simulink library "mbed_targets_stm_nucleo_f303k8"  (R2015a)
settings: Solver=ode45  StartTime=0.0  StopTime=10.0  RelTol=1e-3
libraries: mbed_lib x5
settings Model: CovSFcnEnable=off  Creator=oh  LastModifiedBy=oh
settings DebuggingCC: SolverPrmCheckMsg=warning

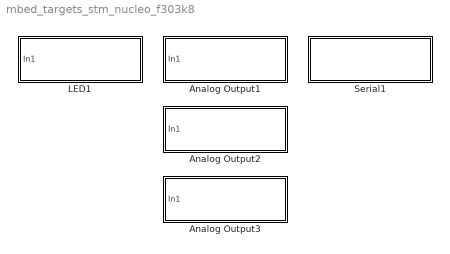
== system mbed_targets_stm_nucleo_f303k8 ==
  Analog Output1 : Subsystem  mask{Parameter1=0}
      mask Display:
      | offset=0.7;
      | plot([0+offset:0.025:0.25+offset],0.3*sin(2*pi*[0:0.1:1])+0.5)
      | port_label('input',1,['DAC1_1 (PA_4)']);
  Analog Output2 : Subsystem  mask{Parameter1=0}
      mask Display:
      | offset=0.7;
      | plot([0+offset:0.025:0.25+offset],0.3*sin(2*pi*[0:0.1:1])+0.5)
      | port_label('input',1,['DAC1_2 (PA_5)']);
  Analog Output3 : Subsystem  mask{Parameter1=0}
      mask Display:
      | offset=0.7;
      | plot([0+offset:0.025:0.25+offset],0.3*sin(2*pi*[0:0.1:1])+0.5)
      | port_label('input',1,['DAC2_1 (PA_6)']);
  LED1 : Subsystem  mask{Parameter1=0}
      mask Display:
      | plot([0.5 0.65 0.65 0.85 0.85 1],[0.3 0.3 0.7 0.7 0.3 0.3])
      | port_label('input',1,['LED1']);
  Serial1 : Subsystem  mask(mbed Serial Configuration){Parameter1=0, BaudRate=9600}
      mask prompts: BaudRate "Baud Rate:"
      mask help:
      | This blocks sets up the serial connection over ST-Link on the NUCLEO_F303 mbed board. You must have one of these blocks in any model that ues the Serial Write or Serial Read blocks.
      |
      | Set the baud rate to match the device that you are communicating with. Standard rates include:300, 1200, 2400, 4800, 9600, 14400, 19200, 28800, 38400, 57600, or 115200.
      mask TypeOptions BaudRate: Serial Configuration/BaudRate
      mask Display: disp(['Serial1(USB)\nTX:PA_2, RX:PA_15'])

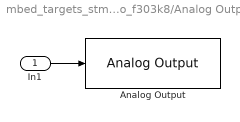
== system mbed_targets_stm_nucleo_f303k8/Analog Output1 ==
  In1 : Inport
  Analog Output : mbed_lib/GPIO/Analog Output  SParameter2=A  SParameter1=4  inputVariant=Double: 0 - 1.0f  SampleTime=-1
  wires:
  In1/1 -> Analog Output/1

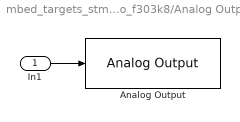
== system mbed_targets_stm_nucleo_f303k8/Analog Output2 ==
  In1 : Inport
  Analog Output : mbed_lib/GPIO/Analog Output  SParameter2=A  SParameter1=5  inputVariant=Double: 0 - 1.0f  SampleTime=-1
  wires:
  In1/1 -> Analog Output/1

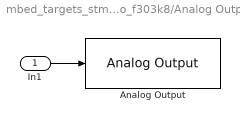
== system mbed_targets_stm_nucleo_f303k8/Analog Output3 ==
  In1 : Inport
  Analog Output : mbed_lib/GPIO/Analog Output  SParameter2=A  SParameter1=6  inputVariant=Double: 0 - 1.0f  SampleTime=-1
  wires:
  In1/1 -> Analog Output/1

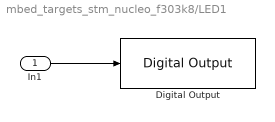
== system mbed_targets_stm_nucleo_f303k8/LED1 ==
  In1 : Inport
  Digital Output : mbed_lib/GPIO/Digital Output  SParameter2=B  SParameter1=3  SParameter3=PullDefault  SampleTime=-1
  wires:
  In1/1 -> Digital Output/1

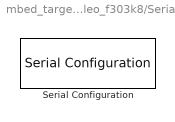
== system mbed_targets_stm_nucleo_f303k8/Serial1 ==
  Serial Configuration : mbed_lib/Serial/Serial Configuration  SerialPort=1  TXPort=A  TXPin=2  RXPort=A  RXPin=15  BaudRate=BaudRate
